simulink model "simModel2020"  (R2023b)
settings: Solver=ode4  StartTime=0  StopTime=360  FixedStep=0.01  RelTol=1e-3
values from neighbouring files (symbols this model uses):
  B747 =     [B747.mat]
undefined symbols (not defined in the file or in its folder): airport, APP, control, Curise, Earth, env, ft, m, navData, navParam, Newton, plotTrack, Raphson, s, TakeOff, WGS84
libraries: aerolibconvert2 x18, simulink x15, sharedtransform x4, aerolibfltsims x3, aerolibatmos2 x2, shared6dof x2, aerolibasang x2, dspsrcs4 x2, aerolibwind2 x2, aerolibanimutils x1, aerolibpropulsion2 x1, aerolibtransform2 x1
(part 6 of 6)

== system simModel2020/PlantModel/B747 Dynamics动力学参数计算/Forces and Moments动力学计算/Compute Body Frame Forces and Moments气动力和力矩/Wind frame F& M 气动力计算/Longitudinal Channel/CL/Lift due to pitch rate ==
  p,q,r : Inport
  Airspeed : Inport  Port=2
  Constant : Constant  Value=B747.aero.CLq
      settings: AttributesFormatString=%<Value>
  Get q : Selector  InputPortWidth=3  IndexOptions=Index vector (dialog)  Indices=2  OutputSizes=[(-2)]
  Product : Product  SaturateOnIntegerOverflow=on  OutDataTypeStr=Inherit: Same as first input
  pitch rate factor : Subsystem
  CLq : Outport
  wires:
  Airspeed/1 -> pitch rate factor/2(Airspeed)
  Get q/1 -> pitch rate factor/1(q)
  p,q,r/1 -> Get q/1
  Product/1 -> CLq/1
  pitch rate factor/1(Pitch Rate Fac) -> Product/2
  Constant/1 -> Product/1

== system simModel2020/PlantModel/B747 Dynamics动力学参数计算/Forces and Moments动力学计算/Compute Body Frame Forces and Moments气动力和力矩/Wind frame F& M 气动力计算/Longitudinal Channel/CL/Subsystem ==
  alpha : Inport
  CLa1 : Constant
      settings: AttributesFormatString=%<Value>
  CLa2 : Constant  Value=B747.aero.alpha0
      settings: AttributesFormatString=%<Value>
  CLa3 : Constant  Value=50
      settings: AttributesFormatString=%<Value>
  CLa4 : Constant  Value=-50
      settings: AttributesFormatString=%<Value>
  CLa5 : Constant
      settings: AttributesFormatString=%<Value>
  Divide : Product  Inputs=*/
  Math Function : Math  SignedPower=on
  Math Function1 : Math  SignedPower=on
  Product : Product
  Product3 : Product
  Product5 : Product
  Sum1 : Sum  Inputs=+-
  Sum2 : Sum
  Sum3 : Sum  Inputs=+++
  Sum4 : Sum  Inputs=++|
  Sum5 : Sum  Inputs=++|
  sigmod : Outport
  wires:
  CLa5/1 -> Sum5/2, Sum4/2
  Sum4/1 -> Product5/1
  Sum5/1 -> Product5/2
  Math Function/1 -> Sum3/2, Sum4/1
  Sum3/1 -> Divide/1
  Product5/1 -> Divide/2
  CLa2/1 -> Sum1/2, Sum2/2
  CLa4/1 -> Product/2
  CLa1/1 -> Sum3/1
  Product/1 -> Math Function/1
  Sum1/1 -> Product/1
  Sum2/1 -> Product3/1
  Math Function1/1 -> Sum3/3, Sum5/1
  Product3/1 -> Math Function1/1
  CLa3/1 -> Product3/2
  Divide/1 -> sigmod/1
  alpha/1 -> Sum2/1, Sum1/1

== system simModel2020/PlantModel/B747 Dynamics动力学参数计算/Forces and Moments动力学计算/Compute Body Frame Forces and Moments气动力和力矩/Wind frame F& M 气动力计算/Longitudinal Channel/Cm/Lift due to pitch rate ==
  p,q,r : Inport
  Airspeed : Inport  Port=2
  Cma1 : Constant  Value=B747.aero.Cmq
      settings: AttributesFormatString=%<Value>
  Get q : Selector  InputPortWidth=3  IndexOptions=Index vector (dialog)  Indices=2  OutputSizes=[(-2)]
  Product : Product  SaturateOnIntegerOverflow=on  OutDataTypeStr=Inherit: Same as first input
  pitch rate factor : Subsystem
  CMq : Outport
  wires:
  Airspeed/1 -> pitch rate factor/2(Airspeed)
  Get q/1 -> pitch rate factor/1(q)
  p,q,r/1 -> Get q/1
  Product/1 -> CMq/1
  pitch rate factor/1(Pitch Rate Fac) -> Product/2
  Cma1/1 -> Product/1

== system simModel2020/PlantModel/B747 Dynamics动力学参数计算/Forces and Moments动力学计算/Compute Body Frame Forces and Moments气动力和力矩/Wind frame F& M 气动力计算/Lateral Channel/Cl/roll factors/roll rate fact ==
  p : Inport
  Airspeed : Inport  Port=2
  Cmq1 : Constant  Value=.5
      settings: AttributesFormatString=%<Value>
  Cmq2 : Constant  Value=B747.geometry.span
      settings: AttributesFormatString=%<Value>
  Product : Product  Inputs=***/  SaturateOnIntegerOverflow=on  OutDataTypeStr=Inherit: Same as first input
  Saturation : Saturate  UpperLimit=inf  LowerLimit=0.1
      settings: AttributesFormatString="[%<LowerLimit>  %<UpperLimit>]"
  Roll Rate Fac : Outport
  wires:
  Saturation/1 -> Product/4
  Airspeed/1 -> Saturation/1
  Cmq2/1 -> Product/3
  Cmq1/1 -> Product/2
  p/1 -> Product/1
  Product/1 -> Roll Rate Fac/1

== system simModel2020/PlantModel/B747 Dynamics动力学参数计算/Forces and Moments动力学计算/Compute Body Frame Forces and Moments气动力和力矩/Wind frame F& M 气动力计算/Lateral Channel/Cl/roll factors/yaw rate fact ==
  r : Inport
  Airspeed : Inport  Port=2
  Cmq3 : Constant  Value=.5
      settings: AttributesFormatString=%<Value>
  Cmq4 : Constant  Value=B747.geometry.span
      settings: AttributesFormatString=%<Value>
  Product1 : Product  Inputs=***/  SaturateOnIntegerOverflow=on  OutDataTypeStr=Inherit: Same as first input
  Saturation : Saturate  UpperLimit=inf  LowerLimit=0.1
      settings: AttributesFormatString="[%<LowerLimit>  %<UpperLimit>]"
  Yaw Rate Fac : Outport
  wires:
  Product1/1 -> Yaw Rate Fac/1
  r/1 -> Product1/1
  Cmq3/1 -> Product1/2
  Cmq4/1 -> Product1/3
  Airspeed/1 -> Saturation/1
  Saturation/1 -> Product1/4

== system simModel2020/PlantModel/B747 Dynamics动力学参数计算/Forces and Moments动力学计算/Compute Body Frame Forces and Moments气动力和力矩/Wind frame F& M 气动力计算/Lateral Channel/Cn/yaw factors/roll rate fact ==
  p : Inport
  Airspeed : Inport  Port=2
  Cmq1 : Constant  Value=.5
      settings: AttributesFormatString=%<Value>
  Cmq2 : Constant  Value=B747.geometry.span
      settings: AttributesFormatString=%<Value>
  Product : Product  Inputs=***/  SaturateOnIntegerOverflow=on  OutDataTypeStr=Inherit: Same as first input
  Saturation : Saturate  UpperLimit=inf  LowerLimit=0.1
      settings: AttributesFormatString="[%<LowerLimit>  %<UpperLimit>]"
  Roll Rate Fac : Outport
  wires:
  Saturation/1 -> Product/4
  Airspeed/1 -> Saturation/1
  Cmq2/1 -> Product/3
  Cmq1/1 -> Product/2
  p/1 -> Product/1
  Product/1 -> Roll Rate Fac/1

== system simModel2020/PlantModel/B747 Dynamics动力学参数计算/Forces and Moments动力学计算/Compute Body Frame Forces and Moments气动力和力矩/Wind frame F& M 气动力计算/Lateral Channel/Cn/yaw factors/yaw rate fact ==
  r : Inport
  Airspeed : Inport  Port=2
  Cmq3 : Constant  Value=.5
      settings: AttributesFormatString=%<Value>
  Cmq4 : Constant  Value=B747.geometry.span
      settings: AttributesFormatString=%<Value>
  Product1 : Product  Inputs=***/  SaturateOnIntegerOverflow=on  OutDataTypeStr=Inherit: Same as first input
  Saturation : Saturate  UpperLimit=inf  LowerLimit=0.1
      settings: AttributesFormatString="[%<LowerLimit>  %<UpperLimit>]"
  Yaw Rate Fac : Outport
  wires:
  Product1/1 -> Yaw Rate Fac/1
  r/1 -> Product1/1
  Cmq3/1 -> Product1/2
  Cmq4/1 -> Product1/3
  Airspeed/1 -> Saturation/1
  Saturation/1 -> Product1/4

== system simModel2020/PlantModel/B747 Dynamics动力学参数计算/Forces and Moments动力学计算/Compute Body Frame Forces and Moments气动力和力矩/Wind frame F& M 气动力计算/Longitudinal Channel/CL/Lift due to pitch rate/pitch rate factor ==
  q : Inport
  Airspeed : Inport  Port=2
  Cmq2 : Constant  Value=B747.geometry.chord
      settings: AttributesFormatString=%<Value>
  Constant : Constant  Value=2
  Product : Product  Inputs=**//  SaturateOnIntegerOverflow=on  OutDataTypeStr=Inherit: Same as first input
  Saturation : Saturate  UpperLimit=inf  LowerLimit=0.1
      settings: AttributesFormatString="[%<LowerLimit>  %<UpperLimit>]"
  Pitch Rate Fac : Outport
  wires:
  Saturation/1 -> Product/3
  Cmq2/1 -> Product/2
  Airspeed/1 -> Saturation/1
  q/1 -> Product/1
  Product/1 -> Pitch Rate Fac/1
  Constant/1 -> Product/4

== system simModel2020/PlantModel/B747 Dynamics动力学参数计算/Forces and Moments动力学计算/Compute Body Frame Forces and Moments气动力和力矩/Wind frame F& M 气动力计算/Longitudinal Channel/Cm/Lift due to pitch rate/pitch rate factor ==
  q : Inport
  Airspeed : Inport  Port=2
  Cmq2 : Constant  Value=B747.geometry.chord
      settings: AttributesFormatString=%<Value>
  Constant : Constant  Value=2
  Product : Product  Inputs=**//  SaturateOnIntegerOverflow=on  OutDataTypeStr=Inherit: Same as first input
  Saturation : Saturate  UpperLimit=inf  LowerLimit=0.1
      settings: AttributesFormatString="[%<LowerLimit>  %<UpperLimit>]"
  Pitch Rate Fac : Outport
  wires:
  Saturation/1 -> Product/3
  Cmq2/1 -> Product/2
  Airspeed/1 -> Saturation/1
  q/1 -> Product/1
  Product/1 -> Pitch Rate Fac/1
  Constant/1 -> Product/4

== matlab function simModel2020/PlantModel/B747 Dynamics动力学参数计算/Forces and Moments动力学计算/Touch the Ground Detection/TakeOff And Landing ==
  settings: updateMethod=DISCRETE
  data: Pos input; v input; Mb input; MbOut output; Pos_ZLXY input; Pos_ZBAA input; TakeOffSpeed input; Ta output; La output
function [MbOut,Ta,La] = fcn(Pos,v,Mb,Pos_ZLXY,Pos_ZBAA,TakeOffSpeed)
Pos_ZLXY(3) = -Pos_ZLXY(3);
Pos_ZBAA(3) = -Pos_ZBAA(3);
MbOut = Mb;
Ta = false;  La = false;
if norm(Pos-Pos_ZLXY) < 3500
 %   a = Pos(3) + Pos_ZLXY(3);
 if (-Pos(3)) <= Pos_ZLXY(3)+0.01
    if  (v < TakeOffSpeed) || (MbOut(2)<0)
        MbOut = [0;0;0];
        Ta = true;
    end
 end

elseif norm(Pos-Pos_ZBAA) < 3500
    b = Pos(3) + Pos_ZBAA(3);
    if b >= 0
        La = true;
        MbOut = [0;0;0];
    end
end

== matlab function simModel2020/Auto_Pilot_Set/Trajectory/MATLAB Function ==
  settings: updateMethod=DISCRETE
  data: t input; WPIndex output; InitialIndex input; FlightLineSeg input; FlightCircleSeg input; FQParam input; WPType output; LLA input; Turn output
function [WPIndex,WPType,Turn] = CurrentRoute( t,InitialIndex,FlightLineSeg,FlightCircleSeg,FQParam,LLA)
%turn == -1  左转
%turn == 1  右转
persistent indexIn;
persistent typeIn;
persistent IndexMax;
if t==0
    typeIn = 1; % 直线
    indexIn = InitialIndex; % 初始一定为直线航段
    IndexMax = size(FlightLineSeg,1);
end
if isempty(typeIn) %判断是否为空，逻辑函数
    typeIn = 1; % 直线
    indexIn = InitialIndex; % 初始一定为直线航段
    IndexMax = size(FlightLineSeg,1);
end
Turn = 0;
if indexIn < IndexMax - 0.1
    if typeIn==1 % 直线
        Pos = LLA(1:2); % 当前位置
        WPC  = FlightCircleSeg(indexIn*2-1,[1,2]);% 对应圆弧的第一个航点
        kai1 = FlightLineSeg(indexIn,5);% 航段航迹角
        kai2 = fanjie(FQParam,Pos,WPC);
        % 计算两航向的夹角
        if abs(kai1-kai2)<180
            delta_kai = abs(kai1-kai2);
        else
            delta_kai = 360-abs(kai1-kai2);
        end
        if delta_kai > 90 % 如果两者角度差大于90度
            typeIn = 0;
        end
    else % 此时为圆弧航段
        Turn = FlightCircleSeg(indexIn*2,4);
        Pos = LLA(1:2); % 当前位置
        WPC  = FlightCircleSeg(indexIn*2,[1,2]);% 对应圆弧的第二个航点
        kai1 = fanjie(FQParam,Pos,WPC);
        kai2 = FlightLineSeg(indexIn+1,5);% 航段航迹角
        % 计算两航向的夹角
        if abs(kai1-kai2)<180
            delta_kai = abs(kai1-kai2);
        else
            delta_kai = 360-abs(kai1-kai2);
        end
        if delta_kai > 90 % 如果两者角度差大于90度
            typeIn = 1;
            indexIn = indexIn + 1;
        end
    end
end
WPIndex = indexIn;
WPType = typeIn;
end

function [kai_rh,S_rh] = fanjie(FQParam, WP1,WP2)
%等角航线的反解
%输入
% L1，lambda1,H1:起始点纬度、经度、高度（deg,deg,m）
% L2，lambda2,H2:终点纬度、经度、高度(deg,deg,m)

%输出
%kai_rh:航向角（deg）
%S_rh:航线长度（nm）
L1 = WP1(1);lambda1 = WP1(2);
L2 = WP2(1);lambda2 = WP2(2);
% 参数
nav.d2r = FQParam(1);
nav.r2d = FQParam(2);
nav.Re  = FQParam(3);
nav.Rp  = FQParam(4);
nav.RL  = FQParam(5);
nav.e   = FQParam(6);
nav.K1  = FQParam(7);
nav.K2  = FQParam(8);
nav.K3  = FQParam(9);
nav.K4  = FQParam(10);
nav.K5  = FQParam(11);

L1 = L1*nav.d2r;
L2 = L2*nav.d2r;
lambda1 = lambda1*nav.d2r;
lambda2 = lambda2*nav.d2r;

%航向角
Lq1 = atanh(sin(L1))-nav.e*atanh(nav.e*sin(L1));
Lq2 = atanh(sin(L2))-nav.e*atanh(nav.e*sin(L2));
if lambda2>=lambda1
    if L2 == L1
        kai_rh = pi/2;
    elseif L2 > L1
        kai_rh = atan((lambda2-lambda1)/(Lq2-Lq1));
    else
        kai_rh = atan((lambda2-lambda1)/(Lq2-Lq1))+pi;
    end
else
    if L2 == L1
        kai_rh = 3*pi/2;
    elseif L2 > L1
        kai_rh = atan((lambda2-lambda1)/(Lq2-Lq1))+2*pi;
    else
        kai_rh = atan((lambda2-lambda1)/(Lq2-Lq1))+pi;
    end
end

%航线长度
if kai_rh == pi/2||kai_rh == 3*pi/2
    N1 = nav.Re/((1-nav.e^2*(sin(L1)^2))^(1/2));
    S_rh = (N1*cos(L1))*(lambda2-lambda1);
else
    X_L1 = nav.Re*(1-nav.e^2)*(nav.K1*L1+nav.K2*sin(2*L1)+nav.K3*sin(4*L1)+nav.K4*sin(6*L1)+nav.K5*sin(8*L1));
    X_L2 = nav.Re*(1-nav.e^2)*(nav.K1*L2+nav.K2*sin(2*L2)+nav.K3*sin(4*L2)+nav.K4*sin(6*L2)+nav.K5*sin(8*L2));
    delta_X = X_L2-X_L1;
    S_rh = delta_X/cos(kai_rh);
end
kai_rh = kai_rh*nav.r2d;
end

== stateflow chart simModel2020/Auto_Pilot_Set/Channel Switch ==
  state TakeOff
    state Departure%离场
      en,du:
      AT_Mode = 3;%推力控制
      Ver_Mode = 2;%滚转保持
      Lat_Mode = 1;%侧向纠偏
      N1_Cmd = 100;%油门
      VS_Cmd = 10;%垂直速率
      Heading_Cmd = Heading_navi;
      fd=3;
    state Taxiing%滑行
      en:
      AT_Mode = 3;
      Ver_Mode = 0;
      Lat_Mode = 0;
      N1_Cmd = 100;
      fd=1;
    state Climb%拉起
      en:
      AT_Mode = 3;%推力控制
      Ver_Mode = 2;%滚转保持
      Lat_Mode = 0;%脱开
      N1_Cmd = 100;%油门
      VS_Cmd = 15;%垂直速率
      fd=2;
    (default) -> Taxiing%滑行
    Taxiing%滑行 -> Climb%拉起 : [IAS>=70]
    Climb%拉起 -> Departure%离场 : [H>=1000]
  state AirlinFlight
    state Climb
      state FisrstClimb
        en:
        AT_Mode = 2;%速度油门控制
        Ver_Mode = 1;%高度保持
        Lat_Mode = 1;%侧向纠偏
        ias_Cmd = 210;
        H_Cmd = 1500;
        Heading_Cmd = Heading_navi;
        du:
        Lat_Mode = 1;%侧向纠偏
        Heading_Cmd = Heading_navi;
        fd=4;
      state SecClimb
        en:
        AT_Mode = 3;%推力控制
        Ver_Mode = 2;%垂直速率控制
        Lat_Mode = 1;%侧向纠偏
        N1_Cmd = 95;
        VS_Cmd = 10;
        Heading_Cmd = Heading_navi;
        du:
        Lat_Mode = 1;
        Heading_Cmd = Heading_navi;
        fd=5;
      state ThirdClimb
        en:
        AT_Mode = 3;%推力控制
        Ver_Mode = 2;%垂直速率控制
        Lat_Mode = 1;%侧向纠偏
        N1_Cmd = 95;
        VS_Cmd = 8;
        Heading_Cmd = Heading_navi;
        du:
        Lat_Mode = 1;
        Heading_Cmd = Heading_navi;
        fd=6;
      state FourthClimb
        en:
        AT_Mode = 3;%推力控制
        Ver_Mode = 2;%垂直速率控制
        Lat_Mode = 1;%侧向纠偏
        N1_Cmd = 95;
        VS_Cmd = 6;
        Heading_Cmd = Heading_navi;
        du:
        Lat_Mode = 1;
        Heading_Cmd = Heading_navi;
        fd=7;
      state RollHlod
        en,du:
        Lat_Mode = 2;%滚转保持
        Roll_Cmd = Roll_navi;
        fd=-1;
      state RollHlod1
        en:
        Lat_Mode = 2;%滚转保持
        Roll_Cmd = Roll_navi;
        du:
        Lat_Mode = 2;%滚转保持
        Roll_Cmd = Roll_navi;
        fd=-1;
      state RollHlod2
        en,du:
        Lat_Mode = 2;%滚转保持
        Roll_Cmd = Roll_navi;
        fd=-1;
      state RollHlod3
        en,du:
        Lat_Mode = 2;%滚转保持
        Roll_Cmd = Roll_navi;
        fd=-1;
      (default) -> FisrstClimb
      FisrstClimb -> SecClimb [order 1] : [IAS>= 200]
      ThirdClimb -> FourthClimb [order 2] : [H >= 6000]
      SecClimb -> ThirdClimb [order 1] : [H >= 4000]
      SecClimb -> AirlinFlight.Climb.RollHlod1 [order 2] : [type == 0]
      AirlinFlight.Climb.RollHlod1 -> SecClimb : [type == 1]
      ThirdClimb -> AirlinFlight.Climb.RollHlod2 [order 1] : [type == 0]
      AirlinFlight.Climb.RollHlod2 -> ThirdClimb : [type == 1]
      FourthClimb -> RollHlod3 : [type == 0]
      RollHlod3 -> FourthClimb : [type == 1]
      FisrstClimb -> AirlinFlight.Climb.RollHlod [order 2] : [type == 0]
      AirlinFlight.Climb.RollHlod -> FisrstClimb : [type == 1]
    state Cruise
      state Cruise
        en:
        AT_Mode = 2;%速度控制
        Ver_Mode = 1;%高度保持
        Lat_Mode = 1;%侧向纠偏
        ias_Cmd = CruiseSpeed;%230
        H_Cmd = CruiseHeight;%8000
        Heading_Cmd = Heading_navi;
        du:
        Lat_Mode = 1;
        Heading_Cmd = Heading_navi;
        fd=8;
      state Cruise1%平飞
        en:
        AT_Mode = 2;
        Ver_Mode = 1;
        Lat_Mode = 1;
        ias_Cmd = CruiseSpeed;
        H_Cmd = CruiseHeight;%8000
        Heading_Cmd = Heading_navi;
        du:
        Lat_Mode = 1;
        Heading_Cmd = Heading_navi;
        fd=9;
      state Cruise12%上升
        en:
        AT_Mode = 2;
        Ver_Mode = 3;
        Lat_Mode = 1;
        Pitch_Cmd=1;
        ias_Cmd = CruiseSpeed;
        du:
        Pitch_Cmd=1;
        ias_Cmd = CruiseSpeed;
        fd=10;
      state Cruise14%恢复
        en:
        AT_Mode = 2;
        Ver_Mode = 1;
        Lat_Mode = 1;
        ias_Cmd = CruiseSpeed;
        H_Cmd = data(WPindex);%8000
        Heading_Cmd = Heading_navi;
        du:
        Lat_Mode = 1;
        Heading_Cmd = Heading_navi;
        fd=11;
      state RollHlod_C14
        en,du:
        Lat_Mode = 2;
        Roll_Cmd = Roll_navi;
        fd=-1;
      state RollHlod_C12
        en,du:
        Lat_Mode = 2;
        Roll_Cmd = Roll_navi;
        fd=-1;
      state RollHlod_C1
        en,du:
        Lat_Mode = 2;
        Roll_Cmd = Roll_navi;
        fd=-1;
      state RollHlod_C2
        en,du:
        Lat_Mode = 2;
        Roll_Cmd = Roll_navi;
        fd=-1;
      (default) -> AirlinFlight.Cruise.Cruise
      AirlinFlight.Cruise.Cruise -> Cruise1%平飞 [order 1] : [WPindex==5]
      Cruise1%平飞 -> Cruise12%上升 [order 1] : [after(1,sec)]
      Cruise12%上升 -> Cruise14%恢复 [order 2] : [after(1,sec)]
      AirlinFlight.Cruise.Cruise -> RollHlod_C1 [order 2] : [type == 0]
      RollHlod_C1 -> AirlinFlight.Cruise.Cruise : [type == 1]
      Cruise1%平飞 -> RollHlod_C2 [order 2] : [type==0]
      RollHlod_C2 -> Cruise1%平飞 : [type == 1]
      Cruise12%上升 -> RollHlod_C12 [order 1] : [type==0]
      RollHlod_C12 -> Cruise12%上升 : [type == 1]
      Cruise14%恢复 -> RollHlod_C14 : [type==0]
      RollHlod_C14 -> Cruise14%恢复 : [type == 1]
    state Decrease
      state LevelFlight2
        %进场高度4000,速度不超过520km/h（144m/s）
        en:
        Ver_Mode = 1;
        H_Cmd = AppHeight;
        IAS0 = IAS;
        en,du:
        AT_Mode = 2;
        ias_Cmd = 130;
        Lat_Mode = 1;
        Heading_Cmd = Heading_navi;
        fd=13;
      state FisrstDecrease
        en:
        AT_Mode = 5;
        Ver_Mode = 2;
        VS_Cmd = -6;
        en,du:
        Lat_Mode = 1;
        Heading_Cmd = Heading_navi;
        fd=12;
      state RollHlod_D2
        en,du:
        Lat_Mode = 2;
        Roll_Cmd = Roll_navi;
        fd=-1;
      state RollHlod_D1
        en,du:
        Lat_Mode = 2;
        Roll_Cmd = Roll_navi;
        fd=-1;
      (default) -> FisrstDecrease
      FisrstDecrease -> LevelFlight2 [order 1] : [H <= AppHeight + 100 ]
      FisrstDecrease -> RollHlod_D1 [order 2] : [type == 0]
      RollHlod_D1 -> FisrstDecrease : [type == 1]
      LevelFlight2 -> RollHlod_D2 : [type == 0]
      RollHlod_D2 -> LevelFlight2 : [type == 1]
    (default) -> Climb
    Climb -> AirlinFlight.Cruise : [H >= CruiseHeight - 100]
    AirlinFlight.Cruise -> Decrease : [K_slope <= -0.01]
  state Approach
    en:
    TurnOverIAF = 0;
    TurnOverIF = 0;
    state To_IAF
      %进场下高减速（下降至2700m）
      en:
      AT_Mode = 5;%怠速
      Ver_Mode = 2;%垂直速率控制
      Lat_Mode = 1;%侧向纠偏
      VS_Cmd = -5;
      Heading_Cmd = Heading_navi;
      du:
      if H<= 2700+100
      Ver_Mode = 1; %高度保持
      H_Cmd = 2700;
      end
      if IAS<= 120
      AT_Mode = 2;%速度控制
      ias_Cmd = 120;
      end
      fd=14;
    state IAF_LocationPoint
      %起始进近，下高减速,2700-1500
      en:
      AT_Mode = 5;
      Ver_Mode = 2;
      Lat_Mode = 1;
      VS_Cmd = -5;
      Heading_Cmd = Heading_navi;
      du:
      if H<= 1500+100
      Ver_Mode = 1; H_Cmd = 1500;
      end
      if IAS<= 100
      AT_Mode = 2; ias_Cmd = 100;
      end
      fd=15;
    state IF_FAF
      en:
      AT_Mode = 2;
      Ver_Mode = 2;
      Lat_Mode = 1;
      ias_Cmd = 90;
      VS_Cmd = -8;
      Heading_Cmd = Heading_navi;
      du:
      if H<= 1200+50
      Ver_Mode = 1; H_Cmd = 1200;
      end
      fd=16;
    state RollHlod2
      en,du:
      Lat_Mode = 2;
      Roll_Cmd = Roll_navi;
      TurnOverIF = 1;
      fd=-1;
    state Flare
      en:
      AT_Mode = 2;%0;
      Lat_Mode = 1;
      ias_Cmd = 80;
      h0 = H;
      du:
      %Ver_Mode = 2;
      %H_Cmd = h0*exp(-(t)/30)+30*(-0.5);
      Ver_Mode = 2;
      VS_Cmd = -1/H+(-0.5);
      fd=18;
    state FinalApproach
      en:
      IAS0 = IAS;
      AT_Mode = 2;
      Ver_Mode = 2;
      Lat_Mode = 1;
      ias_Cmd = 80;
      du:
      VS_Cmd =-IAS*(H-53) / D_PEK;
      Heading_Cmd = Heading_navi;
      fd=17;
    state RollHlod1
      en,du:
      Lat_Mode = 2;
      Roll_Cmd = Roll_navi;
      TurnOverIF = 1;
      fd=-1;
    state RollHlod
      en,du:
      Lat_Mode = 2;%滚转保持
      Roll_Cmd = Roll_navi;
      TurnOverIAF = 1;
      fd=-1;
    (default) -> To_IAF
    IAF_LocationPoint -> IF_FAF [order 1] : [TurnOverIF==1]
    Approach.RollHlod2 -> IF_FAF : [type == 1]
    IF_FAF -> Approach.RollHlod2 [order 2] : [type == 0]
    To_IAF -> IAF_LocationPoint [order 1] : [TurnOverIAF==1]
    IF_FAF -> FinalApproach [order 1] : [D_PEK<=FAF_PEK]
    IAF_LocationPoint -> Approach.RollHlod1 [order 2] : [type == 0]
    Approach.RollHlod1 -> IAF_LocationPoint : [type == 1]
    To_IAF -> Approach.RollHlod [order 2] : [type == 0]
    Approach.RollHlod -> To_IAF : [type == 1]
    FinalApproach -> Flare : [H<=Apph+15]
  (default) -> TakeOff
  TakeOff -> AirlinFlight : [H>=1500]
  AirlinFlight -> Approach : [D_IAF<=20*1852]
  data: WPindex input; ias_Cmd output; H_Cmd output; N1_Cmd output; Heading_navi input; Roll_navi input; type input; K_slope input; H input; IAS input; Psi input; D_IAF input; D_PEK input; CruiseHeight input; CruiseSpeed input; Heading_Cmd output; VS_Cmd output; Roll_Cmd output; AT_Mode output; Ver_Mode output; Lat_Mode output; Pitch_Cmd output; h0 local; AppHeight input; Apph input; IAS0 local; TurnOverIAF local; TurnOverIF local; FAF_PEK input; data input; fd output

== matlab function simModel2020/PlantModel/B747 Dynamics动力学参数计算/Forces and Moments动力学计算/Touch the Ground Detection/Touch the Ground Test ==
  data: y_x output; y_y output; F_x input; F_y input; F_z input; v input; Pos input; y_z output; Pos_ZLXY input; Pos_ZBAA input
function [y_x,y_y,y_z] = fcn(F_x,F_y,F_z,v,Pos,Pos_ZLXY,Pos_ZBAA)
Pos_ZLXY(3) = -Pos_ZLXY(3);
Pos_ZBAA(3) = -Pos_ZBAA(3);
y_x = F_x;
y_y = F_y;
% 机场触地检测
if norm(Pos-Pos_ZLXY) < 3500 || norm(Pos-Pos_ZBAA) < 3500
    %推力检测
    if abs(F_x) < 1e4
        y_x = 0;
        y_y = 0;
    end
    a = Pos(3) + Pos_ZLXY(3);%距离咸阳机场高度
    b = Pos(3) + Pos_ZBAA(3);%距离首都机场高度
    if ( a >= 0 || b >= 0) && F_z >= 0
        F_z = 0;
        if a>=0 && abs(v)> 0.1
            F_z = -100 * a - 10 * v;
        elseif b >= 0 && abs(v)> 0.1
            F_z = -100 * b - 10 * v;
        end
    end
end
y_z = F_z;

== matlab function simModel2020/Auto_Pilot_Set/Dis/MATLAB Function2 ==
  data: LLA input; IAF input; D_IAF output; PEK input; D_PEK output; FQParam input
function [D_IAF,D_PEK] = DisAPP(LLA,IAF,PEK,FQParam)
WP1 = LLA(1:2);
[~,D_IAF] = fanjie(FQParam, WP1,IAF);
[~,D_PEK] = fanjie(FQParam, WP1,PEK);
end

function [kai_rh,S_rh] = fanjie(FQParam, WP1,WP2)
%等角航线的反解
%输入
% L1，lambda1,H1:起始点纬度、经度、高度（deg,deg,m）
% L2，lambda2,H2:终点纬度、经度、高度(deg,deg,m)

%输出
%kai_rh:航向角（deg）
%S_rh:航线长度（nm）
L1 = WP1(1);lambda1 = WP1(2);
L2 = WP2(1);lambda2 = WP2(2);
% 参数
nav.d2r = FQParam(1);
nav.r2d = FQParam(2);
nav.Re  = FQParam(3);
nav.Rp  = FQParam(4);
nav.RL  = FQParam(5);
nav.e   = FQParam(6);
nav.K1  = FQParam(7);
nav.K2  = FQParam(8);
nav.K3  = FQParam(9);
nav.K4  = FQParam(10);
nav.K5  = FQParam(11);

L1 = L1*nav.d2r;
L2 = L2*nav.d2r;
lambda1 = lambda1*nav.d2r;
lambda2 = lambda2*nav.d2r;

%航向角
Lq1 = atanh(sin(L1))-nav.e*atanh(nav.e*sin(L1));
Lq2 = atanh(sin(L2))-nav.e*atanh(nav.e*sin(L2));
if lambda2>=lambda1
    if L2 == L1 
        kai_rh = pi/2;
    elseif L2 > L1 
        kai_rh = atan((lambda2-lambda1)/(Lq2-Lq1));
    else
        kai_rh = atan((lambda2-lambda1)/(Lq2-Lq1))+pi;
    end
else
    if L2 == L1 
        kai_rh = 3*pi/2;
    elseif L2 > L1 
        kai_rh = atan((lambda2-lambda1)/(Lq2-Lq1))+2*pi;
    else
        kai_rh = atan((lambda2-lambda1)/(Lq2-Lq1))+pi;
    end
end

%航线长度
if kai_rh == pi/2||kai_rh == 3*pi/2
    N1 = nav.Re/((1-nav.e^2*(sin(L1)^2))^(1/2));
    S_rh = (N1*cos(L1))*(lambda2-lambda1);
else
    X_L1 = nav.Re*(1-nav.e^2)*(nav.K1*L1+nav.K2*sin(2*L1)+nav.K3*sin(4*L1)+nav.K4*sin(6*L1)+nav.K5*sin(8*L1));
    X_L2 = nav.Re*(1-nav.e^2)*(nav.K1*L2+nav.K2*sin(2*L2)+nav.K3*sin(4*L2)+nav.K4*sin(6*L2)+nav.K5*sin(8*L2));
    delta_X = X_L2-X_L1;
    S_rh = delta_X/cos(kai_rh);
end
kai_rh = kai_rh*nav.r2d;
end

== matlab function simModel2020/Auto_Pilot_Set/Trajectory/MATLAB Function1 ==
  data: WPIndex input; LatDistance output; WPType input; FlightLineSeg input; FQParam input; LLA input; IAS input; FlightCircleP0 input; Phig output; HeadingCmd output; KSlope output; g input; WayPointAlt input
function [LatDistance,Phig,HeadingCmd,KSlope] = RouteCal( WPIndex,...
    WPType,FlightLineSeg,FQParam,LLA,IAS,FlightCircleP0,g,WayPointAlt)
% 输出缺省值
Phig = 0;
HeadingCmd = FlightLineSeg(WPIndex,5);
if WPType == 1 % 直线航段侧偏距
   LLK = FlightLineSeg(WPIndex,[1,2,5]);
   LL = LLA(1:2);
   LatDistance = LatDistanceLine(LLK,LL);
else % 圆弧航段侧偏距
   LLK = FlightCircleP0(WPIndex,1:3); % 圆弧起点及航向
   LLP0 = FlightCircleP0(WPIndex,4:5); % 圆弧圆心
   Dc = LatDistanceLine(LLK,LLP0);
   LL = LLA(1:2);
   [~,Dl] = fanjie(FQParam, LLP0,LL);
   kai_i = FlightLineSeg(WPIndex,5); % 圆弧起始航向角=直线航向
   kai_f = FlightLineSeg(WPIndex+1,5); % 圆弧结束航向角=下一航段航向
   Turn = FlightCircleP0(WPIndex,7);R = FlightCircleP0(WPIndex,8);
   LatDistance = CircleLatDistance(Dc,Dl,kai_i,kai_f,R);
   Phig = atan(IAS^2 / (g*R)) * Turn * 180/pi + 0.01 * LatDistance;
end
    DAlt = WayPointAlt(WPIndex+1) - WayPointAlt(WPIndex);
    DHorizon = FlightLineSeg(WPIndex,4); % 航段长度
    KSlope = tan(DAlt/DHorizon); % 垂直角度
end

% 根据航点，航向，飞机当前位置计算侧偏距
% 飞机在航段的左侧，侧偏距为正（航段是包含航向的）
function LatDistance = LatDistanceLine(LLK,LL)
    nav.d2r = pi/180;
    nav.RL = 6371393;%正球体半径，m
    L0 =LLK(1)*nav.d2r;  % 航段纬度
    lambda0 = LLK(2)*nav.d2r;
    kai_rh = LLK(3)*nav.d2r; % 航段航向角
    L = LL(1)*nav.d2r;  % 飞机当前纬度
    lambda = LL(2)*nav.d2r;
    if kai_rh == pi/2 || kai_rh == 3*pi/2
        LatDistance = (L-L0)*nav.RL;
    else
        lambda1 = lambda0 + tan(kai_rh)*log(cos(L0)*(1+sin(L))/(cos(L)*(1+sin(L0))));
        PP1 = -(lambda-lambda1)*nav.RL*cos(L);
        LatDistance = PP1*cos(kai_rh);
    end
end

function DeltaDis = CircleLatDistance(Dc,Dl,kai_i,kai_f,R)
kai_i = kai_i*pi/180;
kai_f = kai_f*pi/180;
if Dc<0 && abs(kai_f-kai_i)<pi
    DeltaDis = Dl-R;
elseif Dc>0 && abs(kai_f-kai_i)<pi
     DeltaDis = R-Dl;
elseif Dc>0 && abs(kai_f-kai_i)>pi
    DeltaDis = Dl-R;
else
    DeltaDis = R-Dl;
end
end

function [kai_rh,S_rh] = fanjie(FQParam, WP1,WP2)
%等角航线的反解
%输入
% L1，lambda1,H1:起始点纬度、经度、高度（deg,deg,m）
% L2，lambda2,H2:终点纬度、经度、高度(deg,deg,m)

%输出
%kai_rh:航向角（deg）
%S_rh:航线长度（nm）
L1 = WP1(1);lambda1 = WP1(2);
L2 = WP2(1);lambda2 = WP2(2);
% 参数
nav.d2r = FQParam(1);
nav.r2d = FQParam(2);
nav.Re  = FQParam(3);
nav.Rp  = FQParam(4);
nav.RL  = FQParam(5);
nav.e   = FQParam(6);
nav.K1  = FQParam(7);
nav.K2  = FQParam(8);
nav.K3  = FQParam(9);
nav.K4  = FQParam(10);
nav.K5  = FQParam(11);

L1 = L1*nav.d2r;
L2 = L2*nav.d2r;
lambda1 = lambda1*nav.d2r;
lambda2 = lambda2*nav.d2r;

%航向角
Lq1 = atanh(sin(L1))-nav.e*atanh(nav.e*sin(L1));
Lq2 = atanh(sin(L2))-nav.e*atanh(nav.e*sin(L2));
if lambda2>=lambda1
    if L2 == L1 
        kai_rh = pi/2;
    elseif L2 > L1 
        kai_rh = atan((lambda2-lambda1)/(Lq2-Lq1));
    else
        kai_rh = atan((lambda2-lambda1)/(Lq2-Lq1))+pi;
    end
else
    if L2 == L1 
        kai_rh = 3*pi/2;
    elseif L2 > L1 
        kai_rh = atan((lambda2-lambda1)/(Lq2-Lq1))+2*pi;
    else
        kai_rh = atan((lambda2-lambda1)/(Lq2-Lq1))+pi;
    end
end

%航线长度
if kai_rh == pi/2||kai_rh == 3*pi/2
    N1 = nav.Re/((1-nav.e^2*(sin(L1)^2))^(1/2));
    S_rh = (N1*cos(L1))*(lambda2-lambda1);
else
    X_L1 = nav.Re*(1-nav.e^2)*(nav.K1*L1+nav.K2*sin(2*L1)+nav.K3*sin(4*L1)+nav.K4*sin(6*L1)+nav.K5*sin(8*L1));
    X_L2 = nav.Re*(1-nav.e^2)*(nav.K1*L2+nav.K2*sin(2*L2)+nav.K3*sin(4*L2)+nav.K4*sin(6*L2)+nav.K5*sin(8*L2));
    delta_X = X_L2-X_L1;
    S_rh = delta_X/cos(kai_rh);
end
kai_rh = kai_rh*nav.r2d;
end

== matlab function simModel2020/AutoPilot/InnerLoopAutopilot/Latitudinal Channel维度通道/Lateral Correction/MATLAB Function ==
  data: psi_c input; psi input; Psi_Error output
function Psi_Error = fcn(psi_c,psi)
% 计算过度圆弧对应的圆心角
error = psi_c-psi;
if abs(error)<pi
    delta_psi = abs(error);
    FlagSign = 1;
else
    delta_psi = 2*pi-abs(error);
    FlagSign = -1;
end
Psi_Error = delta_psi * sign(error) * FlagSign;

== matlab function simModel2020/AutoPilot/InnerLoopAutopilot/Latitudinal Channel维度通道/Yaw Select/MATLAB Function ==
  data: psi_c input; psi input; Psi_Error output
function Psi_Error = fcn(psi_c,psi)
% 计算过度圆弧对应的圆心角
error = psi_c-psi;
if abs(error)<pi
    delta_psi = abs(error);
    FlagSign = 1;
else
    delta_psi = 2*pi-abs(error);
    FlagSign = -1;
end
Psi_Error = delta_psi * sign(error) * FlagSign;

== stateflow chart simModel2020/Draw Aircraft/DataOut/Chart ==
  state Data
    en:
    coder.extrinsic('Simulation_Platform','updata1');
    app=Simulation_Platform();
  state APP
    du:
    X=data;
    updata1(app,X);
  (default) -> Data
  Data -> APP
  data: data input; app local; X local; t local

== matlab function simModel2020/Draw Aircraft/DataOut/MATLAB Function ==
  data: V_body input; Va output; alpha_deg output; beta_deg output
function [Va, alpha_deg, beta_deg] = calc_inertial_air_data(V_body)
% CALC_INERTIAL_AIR_DATA 由机体系地速矢量计算惯性大气数据
%
% 输入：
%   V_body   - 机体系地速矢量 [u; v; w]，单位 m/s
%              u: 机体纵轴（向前为正）
%              v: 机体横轴（向右为正）
%              w: 机体竖轴（向下为正）
%
% 输出：
%   Va       - 空速，单位 m/s
%   alpha_deg- 迎角，单位 deg（抬头为正）
%   beta_deg - 侧滑角，单位 deg（右滑为正）
%
% 注：不考虑风速，即认为空速 = 地速

    %% 输入检查
    V_body = V_body(:);   % 强制列向量
    % if length(V_body) ~= 3
    %     error('输入 V_body 必须是 3×1 或 1×3 向量');
    % end

    u = V_body(1);
    v = V_body(2);
    w = V_body(3);

    %% 空速
    Va = sqrt(u^2 + v^2 + w^2);

    %% 防止零速度除零
    if Va < 1e-6
        alpha_deg = 0;
        beta_deg  = 0;
        % warning('空速接近零，迎角与侧滑角输出为 0');
        return;
    end

    %% 迎角 α = atan2(w, u)
    alpha_deg = rad2deg(atan2(w, u));

    %% 侧滑角 β = asin(v / Va)
    beta_deg  = rad2deg(asin(v / Va));

end
